simulink model "SimulinkImplementfile"  (R2024a)
settings: Solver=VariableStepAuto  StartTime=0.0  StopTime=10.0  RelTol=1e-3
libraries: dspfdesign x1
settings Model: Creator=Khalid  LastModifiedBy=Khalid

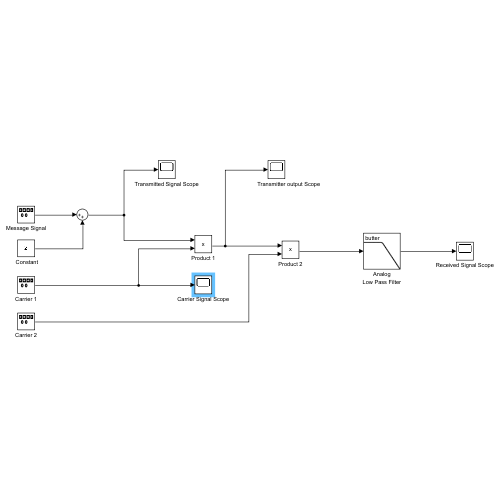
[thumbnail: Simulink's stored preview of the top-level diagram]
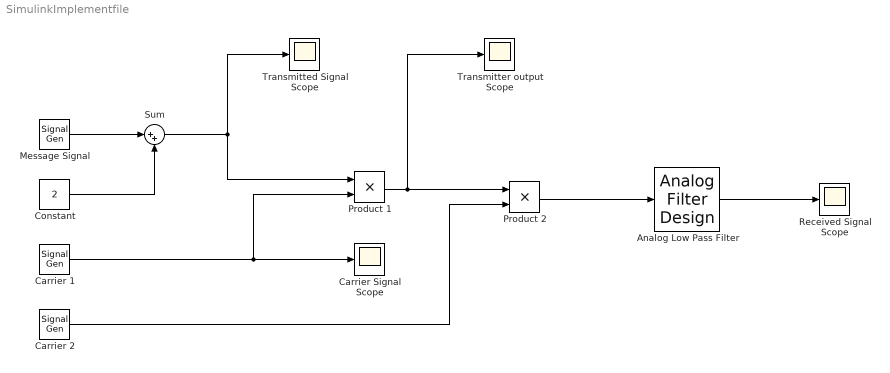
== system SimulinkImplementfile ==
  "                Transmitter output Scope" : Scope
  " Constant" : Constant  Value=2
  Analog Low Pass Filter : dspfdesign/Analog Filter Design  method=Butterworth  filttype=Lowpass  N=8  Wlo=30  Whi=80  Rp=2  Rs=40
  Carrier 1 : SignalGenerator  Frequency=2*pi*10  Units=rad/sec
  Carrier 2 : SignalGenerator  Frequency=2*pi*10  Units=rad/sec
  Carrier Signal Scope : Scope
  Message Signal : SignalGenerator  Frequency=2*pi  Units=rad/sec
  Product 1 : Product
  Product 2 : Product
  Received Signal Scope : Scope
  Sum : Sum  Inputs=|++
  Transmitted Signal Scope : Scope
  wires:
  Message Signal/1 -> Sum/1
  " Constant"/1 -> Sum/2
  Sum/1 -> Transmitted Signal Scope/1, Product 1/1
  Carrier 1/1 -> Product 1/2, Carrier Signal Scope/1
  Product 1/1 -> Product 2/1, "                Transmitter output Scope"/1
  Carrier 2/1 -> Product 2/2
  Product 2/1 -> Analog Low Pass Filter/1
  Analog Low Pass Filter/1 -> Received Signal Scope/1
